simulink model "chuin_krug_model"  (R2023a)
settings: Solver=VariableStepAuto  StartTime=0.0  StopTime=tsim  RelTol=1e-3
values from neighbouring files (symbols this model uses):
  C1 = 1/9    (= 0.111111111111)    [chuin_krug.m]
  C2 = 1    [chuin_krug.m]
  iL0 = 3    [chuin_krug.m]
  L = 1/7    (= 0.142857142857)    [chuin_krug.m]
  R = 1/0.7    (= 1.42857142857)    [chuin_krug.m]
  UC10 = -0.1    [chuin_krug.m]
  UC20 = 0.6    [chuin_krug.m]
  x = [-8, -4, 0, 4, 8]    [chuin_krug.m]
  y = [0, 3.2, 0, -3.2, 0]    [chuin_krug.m]
settings Model: Creator=Vlaho  LastModifiedBy=Enio
settings SolverCC: AlgebraicLoopSolver=TrustRegion
settings DataIOCC: ReturnWorkspaceOutputs=off
settings DebuggingCC: UnconnectedInputMsg=warning  UnconnectedOutputMsg=warning  UnconnectedLineMsg=warning  ArithmeticOperatorsInVariantConditions=warning
settings ModelReferenceCC: EnableRefExpFcnMdlSchedulingChecks=on
settings SFSimCC: SimUseLocalCustomCode=off  CustomCodeUndefinedFunction=UseInterfaceOnly
settings RTWCC: RTWUseLocalCustomCode=off  DLArmComputeVersion=19.05

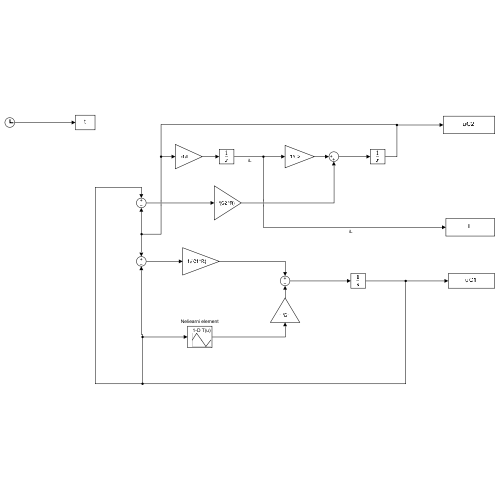
[thumbnail: Simulink's stored preview of the top-level diagram]
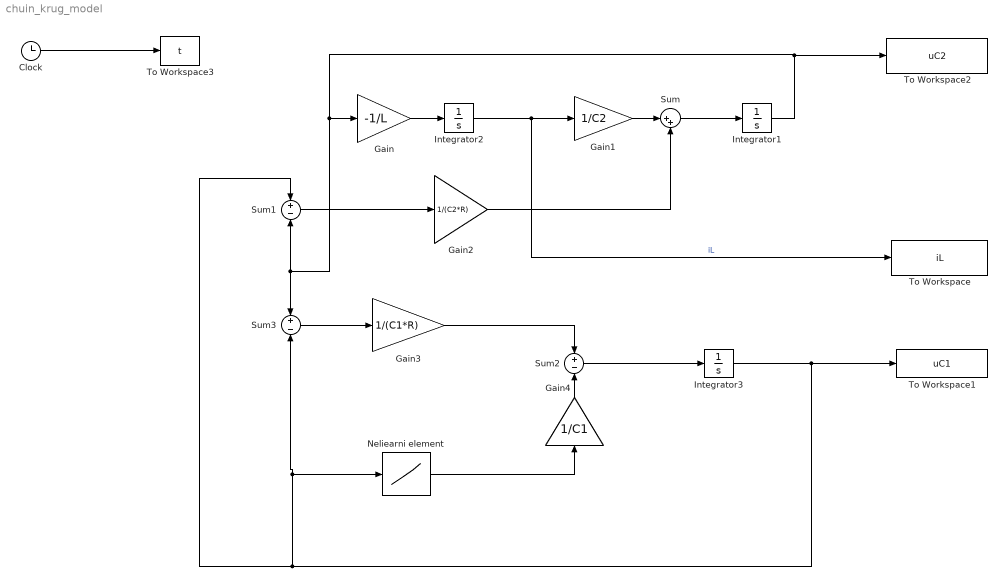
== system chuin_krug_model ==
  Clock : Clock
  Gain : Gain  Gain=-1/L
  Gain1 : Gain  Gain=1/C2
  Gain2 : Gain  Gain=1/(C2*R)
  Gain3 : Gain  Gain=1/(C1*R)
  Gain4 : Gain  Gain=1/C1
  Integrator1 : Integrator  InitialCondition=UC20
  Integrator2 : Integrator  InitialCondition=iL0
  Integrator3 : Integrator  InitialCondition=UC10
  Neliearni element : Lookup_n-D  NumberOfTableDimensions=1  BreakpointsForDimension1=x  Table=y
  Sum : Sum  Inputs=|++
  Sum1 : Sum  Inputs=+-
  Sum2 : Sum  Inputs=+-
  Sum3 : Sum  Inputs=+-
  To Workspace : ToWorkspace  VariableName=iL  SampleTime=0.001
  To Workspace1 : ToWorkspace  VariableName=uC1  SampleTime=0.001
  To Workspace2 : ToWorkspace  VariableName=uC2  SampleTime=0.001
  To Workspace3 : ToWorkspace  VariableName=t  SampleTime=0.001
  wires:
  Gain/1 -> Integrator2/1
  Integrator2/1 -> To Workspace/1, Gain1/1  "iL"
  Gain1/1 -> Sum/1
  Sum1/1 -> Gain2/1
  Gain2/1 -> Sum/2
  Sum/1 -> Integrator1/1
  Integrator1/1 -> Sum1/2, Sum3/1, Gain/1, To Workspace2/1
  Integrator3/1 -> Sum3/2, Neliearni element/1, Sum1/1, To Workspace1/1
  Sum2/1 -> Integrator3/1
  Sum3/1 -> Gain3/1
  Gain3/1 -> Sum2/1
  Gain4/1 -> Sum2/2
  Neliearni element/1 -> Gain4/1
  Clock/1 -> To Workspace3/1
